simulink model "example_of_unit_delay_and_Abs_block"  (R2021a)
settings: Solver=VariableStepAuto  StartTime=0.0  StopTime=10.0  RelTol=1e-3
settings Model: Creator=YasserNet  LastModifiedBy=YasserNet

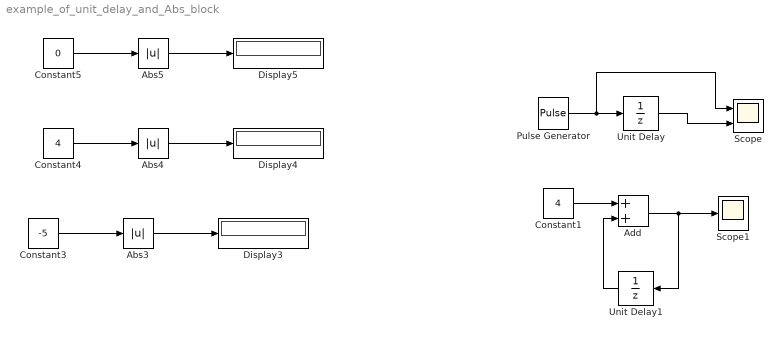
== system example_of_unit_delay_and_Abs_block ==
  Abs3 : Abs
  Abs4 : Abs
  Abs5 : Abs
  Add : Sum
  Constant1 : Constant  Value=4
  Constant3 : Constant  Value=-5
  Constant4 : Constant  Value=4
  Constant5 : Constant  Value=0
  Display3 : Display
  Display4 : Display
  Display5 : Display
  Pulse Generator : DiscretePulseGenerator  PulseType=Time based  PulseWidth=25
  Scope : Scope  NumInputPorts=2
  Scope1 : Scope
  Unit Delay : UnitDelay  SampleTime=-1  HasFrameUpgradeWarning=on
  Unit Delay1 : UnitDelay  SampleTime=-1  HasFrameUpgradeWarning=on
  wires:
  Constant3/1 -> Abs3/1
  Abs3/1 -> Display3/1
  Abs4/1 -> Display4/1
  Constant4/1 -> Abs4/1
  Constant5/1 -> Abs5/1
  Abs5/1 -> Display5/1
  Unit Delay/1 -> Scope/2
  Pulse Generator/1 -> Scope/1, Unit Delay/1
  Add/1 -> Unit Delay1/1, Scope1/1
  Constant1/1 -> Add/1
  Unit Delay1/1 -> Add/2
